simulink model "controllore_simulink"  (Simulink 8.3)
settings: Solver=ode45  StartTime=0.0  StopTime=200  RelTol=1e-3
values from neighbouring files (symbols this model uses):
  D = 1.5    [controllore.m]
  Kr = 1    [controllore.m]
libraries: cstblocks x4, simulink x1
settings Model: Creator=matdo  LastModifiedBy=matdo
settings DataIOCC: SignalLoggingSaveFormat=Dataset
settings DebuggingCC: UnderspecifiedInitializationDetection=Simplified  StateNameClashWarn=none
settings GRTTargetCC: CombineOutputUpdateFcns=on  GRTInterface=off

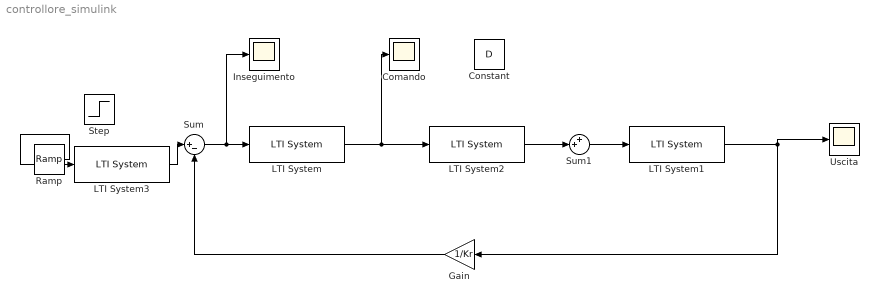
== system controllore_simulink ==
  Comando : Scope
  Constant : Constant  Value=D
  Gain : Gain  Gain=1/Kr
  Inseguimento : Scope
      settings: SaveName=ScopeData2
  LTI System : cstblocks/LTI System  sys=Ci  IC=[]
  LTI System1 : cstblocks/LTI System  sys=F2  IC=[]
  LTI System2 : cstblocks/LTI System  sys=F1  IC=[]
  LTI System3 : cstblocks/LTI System  sys=B  IC=[]
  Ramp : simulink/Sources/Ramp  slope=1  start=0  X0=0
  Step : Step  Time=0  SampleTime=0
  Sum : Sum  Inputs=|+-
  Sum1 : Sum  Inputs=++|
  Uscita : Scope
  wires:
  LTI System2/1 -> Sum1/2
  Sum1/1 -> LTI System1/1
  Sum/1 -> Inseguimento/1, LTI System/1
  LTI System/1 -> Comando/1, LTI System2/1
  LTI System1/1 -> Uscita/1, Gain/1
  Gain/1 -> Sum/2
  LTI System3/1 -> Sum/1
  Ramp/1 -> LTI System3/1
